simulink model "innerControllerTuning"  (R2018a)
settings: Solver=FixedStepAuto  StartTime=0.0  StopTime=20.0  FixedStep=0.005  RelTol=1e-3
values from neighbouring files (symbols this model uses):
  d = 1/2    (= 0.5)    [innerInit.m]    (also in outerInit.m = 0.0024)
  g = 9.81    [innerInit.m]    (also in outerInit.m)
  Ixx = 0.082    [innerInit.m]    (also in outerInit.m = 0.0059)
  Iyy = 0.082    [innerInit.m]    (also in outerInit.m = 0.0059)
  Izz = 0.149    [innerInit.m]    (also in outerInit.m = 0.00116)
  kr = 1/2    (= 0.5)    [innerInit.m]    (also in outerInit.m = 0.1)
  l = 0.315    [innerInit.m]    (also in outerInit.m = 0.255)
  m = 4    [innerInit.m]    (also in outerInit.m = 0.5)
settings Model: Creator=dinies33  LastModifiedBy=giuseppe

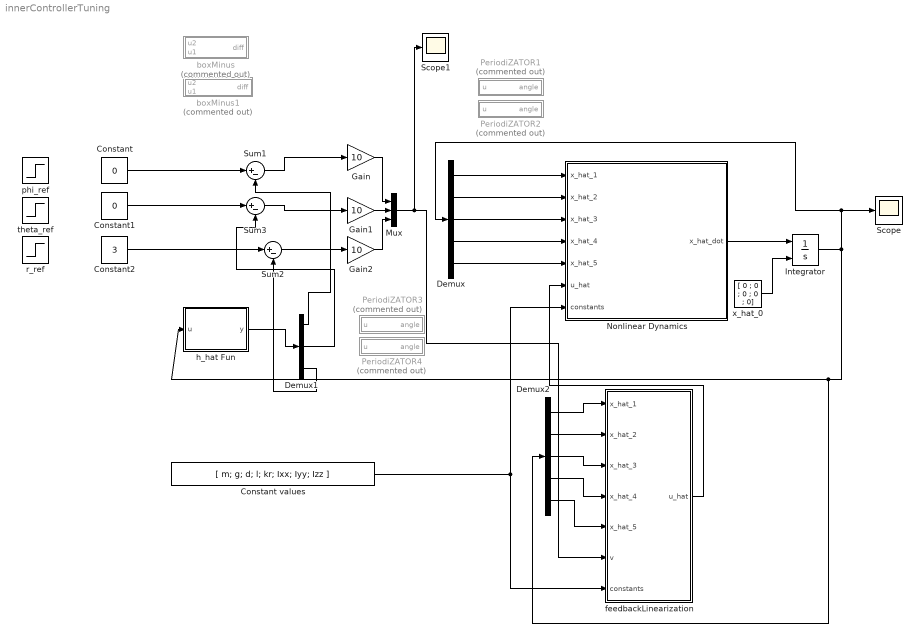
== system innerControllerTuning ==
  Constant : Constant  Value=0
  Constant values : Constant  Value=[ m; g; d; l; kr; Ixx; Iyy; Izz ]
  Constant1 : Constant  Value=0
  Constant2 : Constant  Value=3
  Demux : Demux  Outputs=5
  Demux1 : Demux  Outputs=3
  Demux2 : Demux  Outputs=5
  Gain : Gain  Gain=10
  Gain1 : Gain  Gain=10
  Gain2 : Gain  Gain=10
  Integrator : Integrator  InitialConditionSource=external
  Mux : Mux  Inputs=3
  "Nonlinear Dynamics " : MATLAB Function  TreatAsAtomicUnit=on
  PeriodiZATOR1 : MATLAB Function  Commented=on  TreatAsAtomicUnit=on
  PeriodiZATOR2 : MATLAB Function  Commented=on  TreatAsAtomicUnit=on
  PeriodiZATOR3 : MATLAB Function  Commented=on  TreatAsAtomicUnit=on
  PeriodiZATOR4 : MATLAB Function  Commented=on  TreatAsAtomicUnit=on
  Scope : Scope
  Scope1 : Scope
  Sum1 : Sum  Inputs=|+-
  Sum2 : Sum  Inputs=|+-
  Sum3 : Sum  Inputs=|+-
  boxMinus : MATLAB Function  Commented=on  TreatAsAtomicUnit=on
  boxMinus1 : MATLAB Function  Commented=on  TreatAsAtomicUnit=on
  feedbackLinearization : MATLAB Function  TreatAsAtomicUnit=on
  h_hat Fun : MATLAB Function  TreatAsAtomicUnit=on
  phi_ref : Step  Time=2  After=10  SampleTime=0
  r_ref : Step  SampleTime=0
  theta_ref : Step  SampleTime=0
  x_hat_0 : Constant  Value=[ 0 ; 0 ; 0 ; 0 ; 0]
  wires:
  "Nonlinear Dynamics "/1(x_hat_dot) -> Integrator/1
  x_hat_0/1 -> Integrator/2
  Integrator/1 -> Demux2/1, h_hat Fun/1(u), Demux/1, Scope/1
  h_hat Fun/1(y) -> Demux1/1
  Gain/1 -> Mux/1
  Demux/5 -> "Nonlinear Dynamics "/5(x_hat_5)
  Demux/4 -> "Nonlinear Dynamics "/4(x_hat_4)
  Demux/3 -> "Nonlinear Dynamics "/3(x_hat_3)
  Demux/2 -> "Nonlinear Dynamics "/2(x_hat_2)
  Demux/1 -> "Nonlinear Dynamics "/1(x_hat_1)
  Demux1/1 -> Sum1/2
  Demux1/2 -> Sum3/2
  Demux1/3 -> Sum2/2
  Constant values/1 -> "Nonlinear Dynamics "/7(constants), feedbackLinearization/7(constants)
  Constant/1 -> Sum1/1
  Constant1/1 -> Sum3/1
  Constant2/1 -> Sum2/1
  Gain2/1 -> Mux/3
  Gain1/1 -> Mux/2
  Sum2/1 -> Gain2/1
  Sum3/1 -> Gain1/1
  Sum1/1 -> Gain/1
  Demux2/1 -> feedbackLinearization/1(x_hat_1)
  Demux2/2 -> feedbackLinearization/2(x_hat_2)
  Demux2/3 -> feedbackLinearization/3(x_hat_3)
  Demux2/4 -> feedbackLinearization/4(x_hat_4)
  Demux2/5 -> feedbackLinearization/5(x_hat_5)
  Mux/1 -> Scope1/1, feedbackLinearization/6(v)
  feedbackLinearization/1(u_hat) -> "Nonlinear Dynamics "/6(u_hat)

== matlab function innerControllerTuning/boxMinus1 ==
  data: u2 input; diff output; u1 input
function diff = fcn(u2, u1)

R2 = [cos(u2) -sin(u2);
      sin(u2) cos(u2)];

R1 = [cos(-u1) -sin(-u1);
      sin(-u1) cos(-u1)];

R = R2*R1;

diff = atan2(R(2,1), R(1,1));

== matlab function innerControllerTuning/h_hat Fun ==
  data: u input; y output
function y = fcn(u)

h = [
    1 0 0 0 0;
    0 1 0 0 0;
    0 0 0 0 1;
    ];
    
y = h*u;

== matlab function innerControllerTuning/Nonlinear Dynamics  ==
  data: x_hat_1 input; x_hat_2 input; x_hat_3 input; x_hat_4 input; x_hat_5 input; x_hat_dot output; u_hat input; constants input
function x_hat_dot = fcn(x_hat_1,x_hat_2,x_hat_3,x_hat_4,x_hat_5,u_hat,constants)

m= constants(1,1);
g= constants(2,1);
d= constants(3,1);
l= constants(4,1);
kr= constants(5,1);
Ixx= constants(6,1);
Iyy= constants(7,1);
Izz= constants(8,1);

x_hat = [x_hat_1;
        x_hat_2;
        x_hat_3;
        x_hat_4;
        x_hat_5];

f = [
    x_hat(3,1)+x_hat(4,1)*sin(x_hat(1,1))*tan(x_hat(2,1)) + ( x_hat(5,1)+ m*g*d/kr)*cos(x_hat(1,1))*tan(x_hat(2,1));
    x_hat(4,1)*cos(x_hat(1,1))- (x_hat(5,1)+ m*g*d/kr)*sin(x_hat(1,1)) ;
    1/Ixx*( -kr*x_hat(3,1)- x_hat(4,1)*(x_hat(5,1)+ m*g*d/kr)*(Izz - Ixx));
    1/Iyy*( -kr*x_hat(4,1)- x_hat(3,1)*(x_hat(5,1)+ m*g*d/kr)*(Ixx - Izz));
    1/Izz*(-kr* x_hat(5,1));    
    ];
G = [
    0 , 0 , 0;
    0,  0 , 0;
    l/(2*Ixx), 0 , -l/(2*d*Ixx)
    0,  1/Iyy  , 0 ;
    0 ,  0   ,  1/Izz;
    ];

    
x_hat_dot = f + G*u_hat;

== matlab function innerControllerTuning/PeriodiZATOR2 ==
  data: u input; angle output
function angle = fcn(u)
angle = mod(u, 2*pi);

== matlab function innerControllerTuning/boxMinus ==
  data: u2 input; diff output; u1 input
function diff = fcn(u2, u1)

R2 = [cos(u2) -sin(u2);
      sin(u2) cos(u2)];

R1 = [cos(-u1) -sin(-u1);
      sin(-u1) cos(-u1)];

R = R2*R1;

diff = atan2(R(2,1), R(1,1));

== matlab function innerControllerTuning/PeriodiZATOR3 ==
  data: u input; angle output
function angle = fcn(u)
angle = mod(u, 2*pi);

== matlab function innerControllerTuning/PeriodiZATOR1 ==
  data: u input; angle output
function angle = fcn(u)
angle = mod(u, 2*pi);

== matlab function innerControllerTuning/PeriodiZATOR4 ==
  data: u input; angle output
function angle = fcn(u)
angle = mod(u, 2*pi);

== matlab function innerControllerTuning/feedbackLinearization ==
  data: x_hat_1 input; x_hat_2 input; x_hat_3 input; x_hat_4 input; x_hat_5 input; u_hat output; v input; constants input
function u_hat= fcn(x_hat_1,x_hat_2,x_hat_3,x_hat_4,x_hat_5, v, constants)

m= constants(1,1);
g= constants(2,1);
d= constants(3,1);
l= constants(4,1);
kr= constants(5,1);
Ixx= constants(6,1);
Iyy= constants(7,1);
Izz= constants(8,1);

x1_hat = x_hat_1;
x2_hat = x_hat_2;
x3_hat = x_hat_3;
x4_hat = x_hat_4;
x5_hat = x_hat_5;

alfa = zeros(3,1);

% alfa(1,1) = -2*l*Izz*kr^2*(Ixx*(-1/4*cos(x2)^-2*Izz*(2*d^2*g^2*m^2*...
%     (sin(2*x1) + x1 + cos(2*x2)*(-4*sin(x1) +x1 ) -sin(2*x2)*x2*tan(x1))+...
%     2*d*g*m*kr*( -3*x4 - 4*cos(2*x2)*sin(x1)*x5+ cos(x1)^-1 *(2*x4- ...
%     cos(3*x1)*x4 + 2*cos(2*x1)*cos(2*x2)*x4 + sin(3*x1)*x5)+ ...
%     (2*sin(2*x2)*x3+ x5)* tan(x1))+ kr^2*( -6*x4*x5 - cos(x1)^-1 *...
%     (2 *sin(2*x2)*x3*x4 + 2*cos(3*x1)*x4*x5 + sin(3*x1)*(x4- x5)*(x4+x5))+...
%     (x5^2 - 3*x4^2+2*cos(2*x2)*x4^2)*tan(x1))) - cos(x1)^-1*kr^3*x5*tan(x2))+...
%     Izz*( kr^2*( cos(x1)^-1 *kr*x5*tan(x2) - d*g*m*( x2+ cos(x1)^-1 *(-1+...
%     sin(x1)*x1)*tan(x2)))+Izz*( -kr^2 *x4*x5+d*g*m*kr*(-x4+cos(x1)*x4-...
%     sin(x1)*x5+x3*tan(x1)*tan(x2)+ sin(x1)*( x5+ x4*tan(x1))*tan(x2)^2)+...
%     d^2 * g^2 * m^2 * (x1- x2*tan(x1)*tan(x2)+ sin(x1)* (-1+ tan(x2)^2)))));

% alfa(2,1) =  Izz*kr^2*(Ixx*(-kr^3* x5*tan(x1)+ Izz*( d^2*g^2*m^2*(cos(x1)^-1* ...
%     x2 + (-2+cos(x1)) *tan(x2)) + kr^2*(x3*(2*x5+x4*tan(x1))+ cos(x1)^-1*(sin(x1)*...
%     x4+ cos(x1)*x5)^2 * tan(x2)) + 2*d*g*m*kr*( x3 - cos(x1)^-1*x3+ (sin(x1)*x4- ...
%     x5 +cos(x1)*x5 - x4*tan(x1))* tan(x2)))) + Izz * ( cos(x1)^-1 * kr^2*...
%     (d*g*m*( sin(x1) - x1) + sin(x1)*kr*x5) + Izz *(-kr^2*x3*x5+ d^2*g^2*m^2*...
%     (-cos(x1)^-1*x2 + tan(x2))+ d*g*m*kr*((-1+ cos(x1)^-1)*x3+(x5+x4*tan(x1))*...
%     tan(x2)))));

% alfa(3,1) = 0;

alfa(1,1) = x1_hat*((d*g*m*((2*Ixx*((d*g*m)/kr + (d*g*m*(Ixx - Izz))/(Ixx*kr)))/l + (2*kr*sin(x1_hat)*tan(x2_hat))/(l*cos(x1_hat))))/kr - (2*Ixx*d^2*g^2*m^2)/(kr^2*l)) - (sin(x1_hat)*(x5_hat + (d*g*m)/kr) - x4_hat*cos(x1_hat))*((2*Ixx*((d*g*m)/kr + (d*g*m*(Ixx - Izz))/(Ixx*kr)))/l + (2*kr*sin(x1_hat)*tan(x2_hat))/(l*cos(x1_hat))) + x2_hat*((d*g*m*((2*kr)/l - (2*Ixx*sin(x1_hat)*tan(x2_hat)*((d*g*m)/kr + (d*g*m*(Ixx - Izz))/(Ixx*kr)))/(l*cos(x1_hat))))/kr + (2*Ixx*d^2*g^2*m^2*sin(x1_hat)*tan(x2_hat))/(kr^2*l*cos(x1_hat))) - ((2*kr)/l - (2*Ixx*sin(x1_hat)*tan(x2_hat)*((d*g*m)/kr + (d*g*m*(Ixx - Izz))/(Ixx*kr)))/(l*cos(x1_hat)))*(x3_hat + cos(x1_hat)*tan(x2_hat)*(x5_hat + (d*g*m)/kr) + x4_hat*sin(x1_hat)*tan(x2_hat)) + (2*Ixx*((kr*x3_hat - x4_hat*(x5_hat + (d*g*m)/kr)*(Ixx - Izz))/Ixx + (sin(x1_hat)*tan(x2_hat)*(x5_hat + (d*g*m)/kr) - x4_hat*cos(x1_hat)*tan(x2_hat))*(x3_hat + cos(x1_hat)*tan(x2_hat)*(x5_hat + (d*g*m)/kr) + x4_hat*sin(x1_hat)*tan(x2_hat)) + (sin(x1_hat)*(x5_hat + (d*g*m)/kr) - x4_hat*cos(x1_hat))*(cos(x1_hat)*(x5_hat + (d*g*m)/kr)*(tan(x2_hat)^2 + 1) + x4_hat*sin(x1_hat)*(tan(x2_hat)^2 + 1)) + (sin(x1_hat)*tan(x2_hat)*(kr*x4_hat + x3_hat*(x5_hat + (d*g*m)/kr)*(Ixx - Izz)))/Ixx + (kr*x5_hat*cos(x1_hat)*tan(x2_hat))/Izz))/l - (2*Ixx*sin(x1_hat)*tan(x2_hat)*((cos(x1_hat)*(x5_hat + (d*g*m)/kr) + x4_hat*sin(x1_hat))*(x3_hat + cos(x1_hat)*tan(x2_hat)*(x5_hat + (d*g*m)/kr) + x4_hat*sin(x1_hat)*tan(x2_hat)) + (cos(x1_hat)*(kr*x4_hat + x3_hat*(x5_hat + (d*g*m)/kr)*(Ixx - Izz)))/Ixx - (kr*x5_hat*sin(x1_hat))/Izz))/(l*cos(x1_hat));

alfa(2,1) = (kr*(sin(x1_hat)*(x5_hat + (d*g*m)/kr) - x4_hat*cos(x1_hat)))/cos(x1_hat) - x2_hat*((Ixx*d^2*g^2*m^2)/(kr^2*cos(x1_hat)) - (Ixx*d*g*m*((d*g*m)/kr + (d*g*m*(Ixx - Izz))/(Ixx*kr)))/(kr*cos(x1_hat))) + (Ixx*((cos(x1_hat)*(x5_hat + (d*g*m)/kr) + x4_hat*sin(x1_hat))*(x3_hat + cos(x1_hat)*tan(x2_hat)*(x5_hat + (d*g*m)/kr) + x4_hat*sin(x1_hat)*tan(x2_hat)) + (cos(x1_hat)*(kr*x4_hat + x3_hat*(x5_hat + (d*g*m)/kr)*(Ixx - Izz)))/Ixx - (kr*x5_hat*sin(x1_hat))/Izz))/cos(x1_hat) - (Ixx*((d*g*m)/kr + (d*g*m*(Ixx - Izz))/(Ixx*kr))*(x3_hat + cos(x1_hat)*tan(x2_hat)*(x5_hat + (d*g*m)/kr) + x4_hat*sin(x1_hat)*tan(x2_hat)))/cos(x1_hat) - (d*g*m*x1_hat)/cos(x1_hat);

alfa(3,1) = 0;

% % elem 2,2 is dubious, on the paper is written as SCx1, what is S ?
% beta = [
%     1 , -2*(tan(x1)*tan(x2))/l , -2*(cos(x1)^-1*Ixx*tan(x2))/(l*Izz) ; 
%     0 ,  1/cos(x1) , Ixx*tan(x1)/Izz ;
%     0 ,  0  ,   1;
%     ];

% elem 2,2 is dubious, on the paper is written as SCx1, what is S ?
beta = [
    1, -(2*sin(x1_hat)*sin(x2_hat))/(l*cos(x1_hat)*cos(x2_hat)), -(2*Ixx*sin(x2_hat))/(Izz*l*cos(x1_hat)*cos(x2_hat)) ; 
    0,                                          1/cos(x1_hat),                (Ixx*sin(x1_hat))/(Izz*cos(x1_hat)) ;
    0,                                                       0,                                                  1;
    ];


u_hat = alfa + beta*v;
